simulink model "interpTest"  (R2019a)
settings: Solver=VariableStepAuto  StartTime=0.0  StopTime=10.0  RelTol=1e-3
libraries: simulink x3
settings Model: Creator=first  LastModifiedBy=first

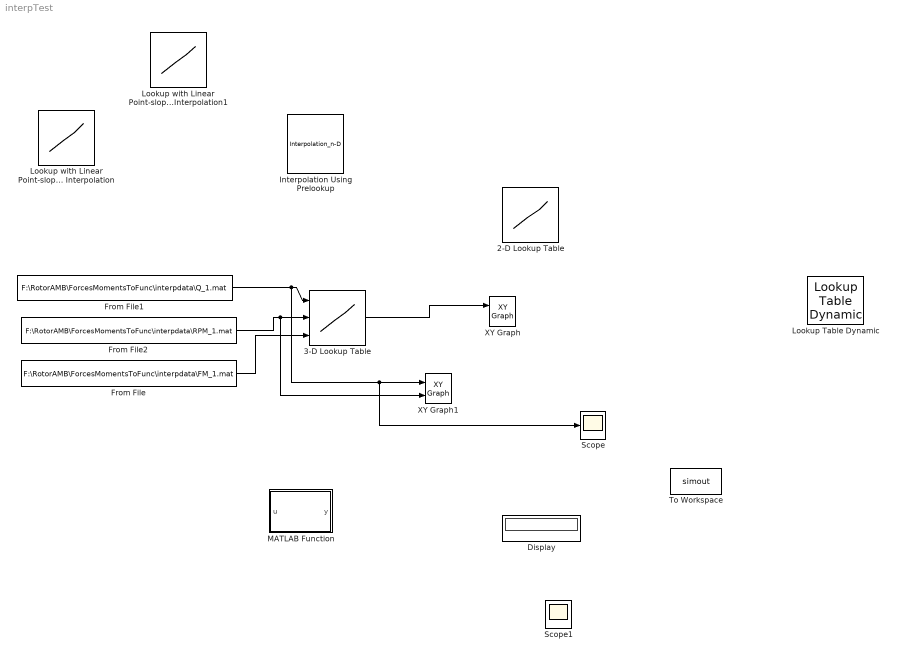
== system interpTest ==
  2-D Lookup Table : Lookup_n-D  BreakpointsForDimension1=[1:3]  BreakpointsForDimension2=[1:3]  InternalRulePriority=Speed  RndMeth=Simplest  InputSameDT=on
  3-D Lookup Table : Lookup_n-D  NumberOfTableDimensions=3  BreakpointsForDimension3=[5, 7]  Table=reshape(repmat([4 5 6;16 19 20;10 18 23],1,2),[3,3,2])  InternalRulePriority=Speed  RndMeth=Simplest  InputSameDT=on
  Display : Display
  From File : FromFile  FileName=F:\RotorAMB\ForcesMomentsToFunc\interpdata\FM_1.mat  SampleTime=0
  From File1 : FromFile  FileName=F:\RotorAMB\ForcesMomentsToFunc\interpdata\Q_1.mat  SampleTime=0
  From File2 : FromFile  FileName=F:\RotorAMB\ForcesMomentsToFunc\interpdata\RPM_1.mat  SampleTime=0
  Interpolation Using Prelookup : Interpolation_n-D  InternalRulePriority=Speed
  Lookup Table Dynamic : simulink/Lookup Tables/Lookup Table Dynamic  LookUpMeth=Interpolation-Use End Values  OutDataType=fixdt('double')  OutScaling=2^-10  OutputDataTypeScalingMode=Specify via dialog  OutDataTypeStr=double  DoSatur=off
      settings: SourceProductName=Simulink
  Lookup with Linear Point-slope Interpolation : Lookup_n-D  NumberOfTableDimensions=1  BreakpointsForDimension1=[-5:5]  Table=tanh([-5:5])  InternalRulePriority=Speed  RndMeth=Simplest  InputSameDT=on
  Lookup with Linear Point-slope Interpolation1 : Lookup_n-D  NumberOfTableDimensions=1  BreakpointsForDimension1=[-5:5]  Table=tanh([-5:5])  InternalRulePriority=Speed  RndMeth=Simplest  InputSameDT=on
  MATLAB Function : MATLAB Function  TreatAsAtomicUnit=on
  Scope : Scope
  Scope1 : Scope  NumInputPorts=3
  To Workspace : ToWorkspace  VariableName=simout  SaveFormat=Timeseries  SampleTime=-1
  XY Graph : simulink/Sinks/XY Graph  xmin=-1  xmax=1  ymin=-1  ymax=1  st=-1
  XY Graph1 : simulink/Sinks/XY Graph  xmin=-1  xmax=1  ymin=-1  ymax=1  st=-1
  wires:
  From File1/1 -> Scope/1, XY Graph1/1, 3-D Lookup Table/1
  From File2/1 -> XY Graph1/2, 3-D Lookup Table/2
  From File/1 -> 3-D Lookup Table/3
  3-D Lookup Table/1 -> XY Graph/1

== matlab function interpTest/MATLAB Function ==
  data: u input; y output
function y = fcn(u)

y = u;
